simulink model "Sliding_Mode_observer"  (R2017a)
settings: Solver=VariableStepAuto  StartTime=0.0  StopTime=10.0  RelTol=1e-3
settings Model: Creator=firass2019  LastModifiedBy=firass2019

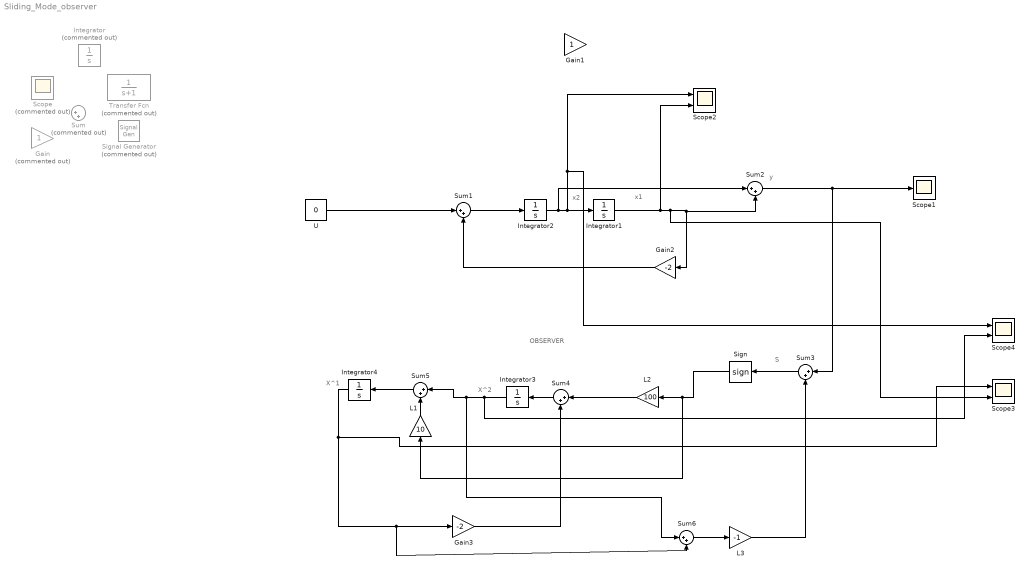
== system Sliding_Mode_observer ==
  note: OBSERVER
  note: X^1
  note: X^2
  note: S
  note: y
  note: x2
  note: x1
  Gain : Gain  Commented=on
  Gain1 : Gain
  Gain2 : Gain  Gain=-2
  Gain3 : Gain  Gain=-2
  Integrator : Integrator  Commented=on
  Integrator1 : Integrator
  Integrator2 : Integrator  InitialCondition=1
  Integrator3 : Integrator  InitialCondition=1
  Integrator4 : Integrator  InitialCondition=1
  L1 : Gain  Gain=10
  L2 : Gain  Gain=100
  L3 : Gain  Gain=-1
  Scope : Scope  Commented=on
  Scope1 : Scope
  Scope2 : Scope  NumInputPorts=2
  Scope3 : Scope  NumInputPorts=2
  Scope4 : Scope  NumInputPorts=2
  Sign : Signum  ZeroCross=off
  Signal Generator : SignalGenerator  Commented=on  Units=rad/sec
  Sum : Sum  Commented=on  Inputs=|++
  Sum{1..6} (6 alike) : Sum  Inputs=|++
  Transfer Fcn : TransferFcn  Commented=on  Denominator=[1 1]
  U : Constant  Value=0
  wires:
  Integrator2/1 -> Sum2/1, Scope4/1, Scope2/1, Integrator1/1
  Integrator1/1 -> Scope2/2, Scope3/2, Sum2/2, Gain2/1
  Sum1/1 -> Integrator2/1
  Sum2/1 -> Sum3/1, Scope1/1
  Gain2/1 -> Sum1/2
  U/1 -> Sum1/1
  Sum3/1 -> Sign/1
  Sign/1 -> L1/1, L2/1
  L2/1 -> Sum4/1
  Sum4/1 -> Integrator3/1
  Integrator3/1 -> Scope4/2, Sum6/1, Sum5/1
  L1/1 -> Sum5/2
  Sum5/1 -> Integrator4/1
  Integrator4/1 -> Scope3/1, Sum6/2, Gain3/1
  Gain3/1 -> Sum4/2
  Sum6/1 -> L3/1
  L3/1 -> Sum3/2
